simulink model "ROMI_FinalModel"  (R2022b)
settings: Solver=FixedStepDiscrete  StartTime=0.0  StopTime=300  FixedStep=0.1  RelTol=1e-3
libraries: nvidiaAVlib x2, dspindex x2, simulink x2, visiontextngfix x1, deeplib x1, visionstatistics x1
settings Model: Creator=HYUH  LastModifiedBy=HYUH
settings OptimizationCC: StrengthReduction=on  PassReuseOutputArgsAs=Individual arguments  ZeroExternalMemoryAtStartup=off  ZeroInternalMemoryAtStartup=off  InitFltsAndDblsToZero=on  MaxStackSize=64  SimCompilerOptimization=on  OptimizeBlockOrder=speed  OptimizationPriority=Speed  EfficientTunableParamExpr=on
settings DebuggingCC: ParameterTunabilityLossMsg=error
settings HardwareCC: ProdBitPerLong=64  ProdLargestAtomicInteger=LongLong  ProdLargestAtomicFloat=Double  ProdLongLongMode=on  ProdHWDeviceType=ARM Compatible->ARM 64-bit (LP64)  TargetLongLongMode=on
settings ModelReferenceCC: EnableRefExpFcnMdlSchedulingChecks=on
settings SFSimCC: SimHardwareAcceleration=native  SimTargetLang=C++  GPUAcceleration=on  SimDLTargetLibrary=cudnn
settings RTWCC: Description=Embedded Coder  SystemTargetFile=ert.tlc  HardwareBoard=NVIDIA Jetson  TLCOptions="-aInlineSetEventsForThisBaseRateFcn=TLC_FALSE -aSuppressMultiTaskScheduler=TLC_FALSE  -aRateBasedStepFcn=0"  TemplateMakefile=ert_default_tmf  Toolchain=NVCC for NVIDIA Embedded Processors  BuildConfiguration=Faster Runs  TargetLang=C++  GenerateGPUCode=CUDA  DLTargetLibrary=cudnn
settings CodeAppCC: ForceParamTrailComments=on  IgnoreCustomStorageClasses=off  OperatorAnnotations=on  SimulinkDataObjDesc=on  SFDataObjDesc=on  InsertBlockDesc=on
settings ERTTargetCC: MatFileLogging=on  SupportVariableSizeSignals=on  ExtModeStaticAlloc=on  RootIOFormat=Structure reference

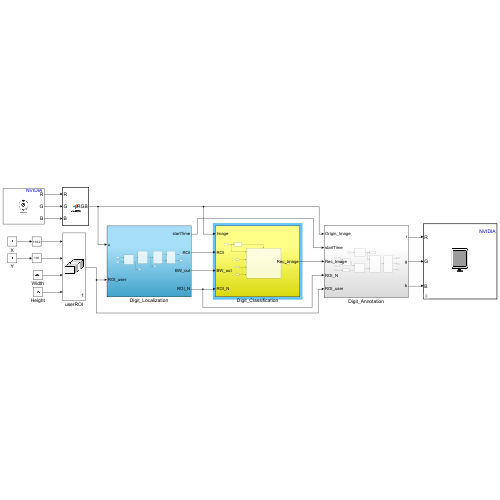
[thumbnail: Simulink's stored preview of the top-level diagram]
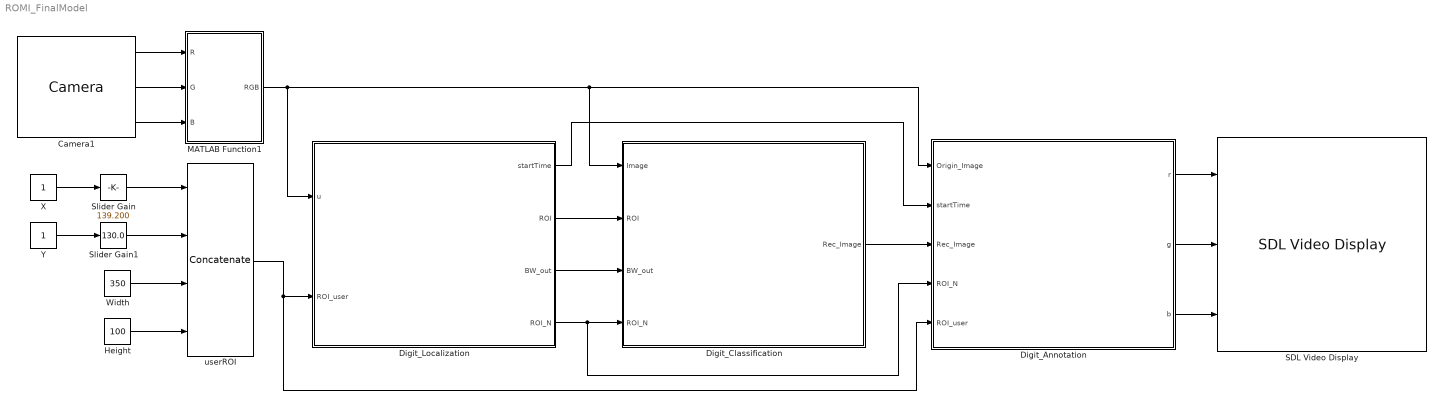
== system ROMI_FinalModel ==
  Camera1 : nvidiaAVlib/Camera  CameraName=UVC Camera (046d:0825)  ImageSize=[640 480]  SampleTime=0.1  SimulateUsing=Code generation
  Digit_Annotation : Subsystem
  Digit_Classification : Subsystem
  Digit_Localization : Subsystem
  Height : Constant  Value=100
  MATLAB Function1 : MATLAB Function  TreatAsAtomicUnit=on
  SDL Video Display : nvidiaAVlib/SDL Video Display  pixelFormat=RGB  pixelOrder=Planar  rowMajor=on  blockPlatform=NVIDIA
  Slider Gain : simulink/Math Operations/Slider Gain  gain=139.200  low=0  high=480
  Slider Gain1 : simulink/Math Operations/Slider Gain  gain=130.0  low=0  high=640
  Width : Constant  Value=350
  X : Constant
  Y : Constant
  userROI : Concatenate  NumInputs=4  Mode=Multidimensional array
  wires:
  Width/1 -> userROI/3
  Height/1 -> userROI/4
  X/1 -> Slider Gain/1
  Y/1 -> Slider Gain1/1
  Camera1/1 -> MATLAB Function1/1(R)
  Camera1/2 -> MATLAB Function1/2(G)
  Camera1/3 -> MATLAB Function1/3(B)
  Slider Gain1/1 -> userROI/2
  Slider Gain/1 -> userROI/1
  MATLAB Function1/1(RGB) -> Digit_Annotation/1(Origin_Image), Digit_Classification/1(Image), Digit_Localization/1(u)
  Digit_Annotation/3(b) -> SDL Video Display/3
  userROI/1 -> Digit_Annotation/5(ROI_user), Digit_Localization/2(ROI_user)
  Digit_Localization/1(startTime) -> Digit_Annotation/2(startTime)
  Digit_Localization/2(ROI) -> Digit_Classification/2(ROI)
  Digit_Localization/3(BW_out) -> Digit_Classification/3(BW_out)
  Digit_Localization/4(ROI_N) -> Digit_Classification/4(ROI_N), Digit_Annotation/4(ROI_N)
  Digit_Classification/1(Rec_Image) -> Digit_Annotation/3(Rec_Image)
  Digit_Annotation/1(r) -> SDL Video Display/1
  Digit_Annotation/2(g) -> SDL Video Display/2

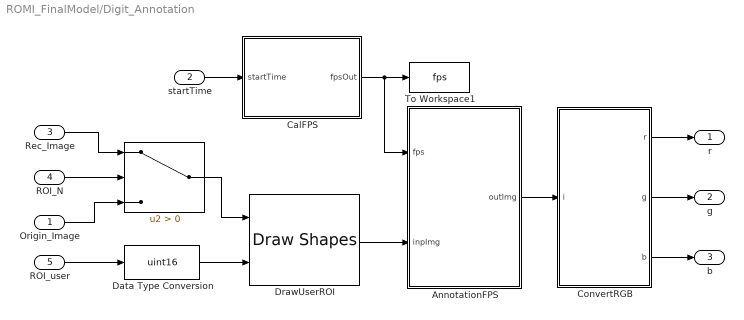
== system ROMI_FinalModel/Digit_Annotation ==
  Origin_Image : Inport
  startTime : Inport  Port=2
  Rec_Image : Inport  Port=3
  ROI_N : Inport  Port=4
  ROI_user : Inport  Port=5
  " " : Switch  Criteria=u2 > Threshold  SaturateOnIntegerOverflow=off  InputSameDT=off
  AnnotationFPS : MATLAB Function  TreatAsAtomicUnit=on
  CalFPS : MATLAB Function  TreatAsAtomicUnit=on
  ConvertRGB : MATLAB Function  TreatAsAtomicUnit=on
  Data Type Conversion : DataTypeConversion  OutDataTypeStr=uint16  SaturateOnIntegerOverflow=off  RndMeth=Floor
  DrawUserROI : visiontextngfix/Draw Shapes  shape=Rectangles  fill=off  lineWidth=3  fillClrSource=Specify via dialog  display=Black  intensity=200  color=[200 255 100]  opacity=0.6  viewport=Entire image  antialiasing=off  inType=Obsolete  imagePorts=One multidimensional signal  roundingMode=Floor  overflowMode=off  memoryMode=Specify word length  memoryWordLength=16  prodOutputMode=Binary point scaling  prodOutputWordLength=32  prodOutputFracLength=14  memoryFracLength=15
  To Workspace1 : ToWorkspace  VariableName=fps  SaveFormat=Structure With Time  SampleTime=-1
  r : Outport
  g : Outport  Port=2
  b : Outport  Port=3
  wires:
  startTime/1 -> CalFPS/1(startTime)
  Rec_Image/1 -> " "/1
  Data Type Conversion/1 -> DrawUserROI/2
  ROI_user/1 -> Data Type Conversion/1
  ROI_N/1 -> " "/2
  Origin_Image/1 -> " "/3
  CalFPS/1(fpsOut) -> To Workspace1/1, AnnotationFPS/1(fps)
  " "/1 -> DrawUserROI/1
  DrawUserROI/1 -> AnnotationFPS/2(inpImg)
  AnnotationFPS/1(outImg) -> ConvertRGB/1(i)
  ConvertRGB/2(g) -> g/1
  ConvertRGB/1(r) -> r/1
  ConvertRGB/3(b) -> b/1

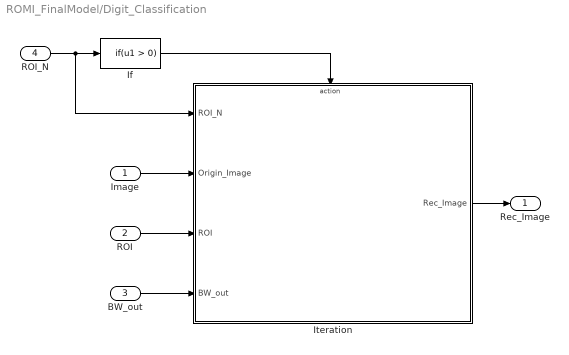
== system ROMI_FinalModel/Digit_Classification ==
  Image : Inport
  ROI : Inport  Port=2
  BW_out : Inport  Port=3
  ROI_N : Inport  Port=4
  If : If  ShowElse=off
  Iteration : Subsystem  TreatAsAtomicUnit=on
  Rec_Image : Outport
  wires:
  Iteration/1(Rec_Image) -> Rec_Image/1
  ROI_N/1 -> If/1, Iteration/1(ROI_N)
  ROI/1 -> Iteration/3(ROI)
  BW_out/1 -> Iteration/4(BW_out)
  Image/1 -> Iteration/2("Origin_Image ")
  If/1 -> Iteration/Action

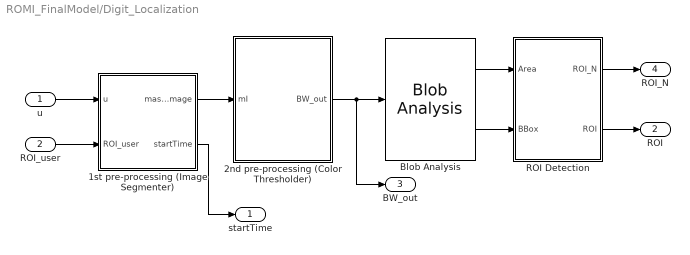
== system ROMI_FinalModel/Digit_Localization ==
  u : Inport
  ROI_user : Inport  Port=2
  1st pre-processing (Image Segmenter) : MATLAB Function  TreatAsAtomicUnit=on
  2nd pre-processing (Color Thresholder) : MATLAB Function  TreatAsAtomicUnit=on
  Blob Analysis : visionstatistics/Blob Analysis  Tag=vipblks_row_conv  area=on  centroid=off  bBox=on  majorAxis=off  minorAxis=off  angle=off  eccentricity=off  equivDiameterSq=off  extent=off  perimeter=off  outDT=double  conn=8  isLabel=off  maxBlobs=50  warnIfNumBlobsExceeded=on  isCount=off  useMinArea=off  minArea=0  useMaxArea=off  maxArea=intmax('uint32')  excludeBorderBlob=off  isOutVarDim=off  isFill=on  fillValues=-1  roundingMode=Floor  overflowMode=off  prodOutputMode=Binary point scaling  prodOutputWordLength=32  prodOutputFracLength=16  accumMode=Binary point scaling  accumWordLength=32  accumFracLength=0  outputMode=Binary point scaling  outputWordLength=32  outputFracLength=16  firstCoeffMode=Binary point scaling  firstCoeffWordLength=16  firstCoeffFracLength=14  secondCoeffMode=Binary point scaling  secondCoeffWordLength=32  secondCoeffFracLength=16
  ROI Detection : MATLAB Function  TreatAsAtomicUnit=on
  startTime : Outport
  ROI : Outport  Port=2
  BW_out : Outport  Port=3
  ROI_N : Outport  Port=4
  wires:
  u/1 -> 1st pre-processing (Image Segmenter)/1(u)
  ROI_user/1 -> 1st pre-processing (Image Segmenter)/2(ROI_user)
  ROI Detection/1(ROI_N) -> ROI_N/1
  Blob Analysis/2 -> ROI Detection/2(BBox)
  2nd pre-processing (Color Thresholder)/1(BW_out) -> BW_out/1, Blob Analysis/1
  1st pre-processing (Image Segmenter)/1(maskedImage) -> 2nd pre-processing (Color Thresholder)/1(mI)
  1st pre-processing (Image Segmenter)/2(startTime) -> startTime/1
  Blob Analysis/1 -> ROI Detection/1(Area)
  ROI Detection/2(ROI) -> ROI/1

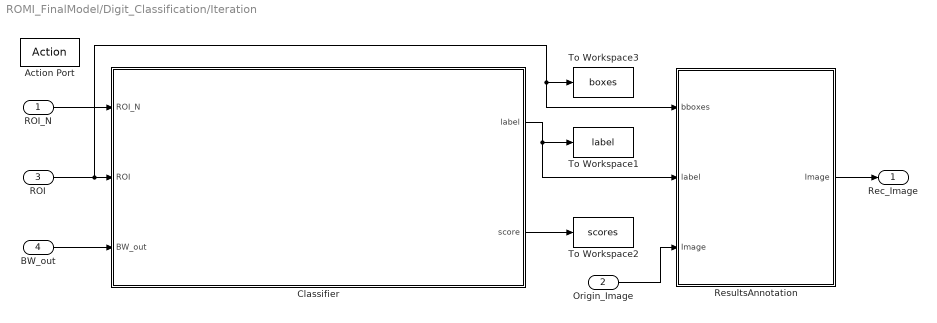
== system ROMI_FinalModel/Digit_Classification/Iteration ==
  ROI_N : Inport
  "Origin_Image " : Inport  Port=2
  ROI : Inport  Port=3
  BW_out : Inport  Port=4
  Action Port : ActionPort  PropagateVarSize=During execution  ActionPortLabel=if(u1 > 0)
  Classifier : Subsystem  TreatAsAtomicUnit=on
  ResultsAnnotation : MATLAB Function  TreatAsAtomicUnit=on
  To Workspace1 : ToWorkspace  VariableName=label  SaveFormat=Structure With Time  SampleTime=-1
  To Workspace2 : ToWorkspace  VariableName=scores  SaveFormat=Structure With Time  SampleTime=-1
  To Workspace3 : ToWorkspace  VariableName=boxes  SaveFormat=Structure With Time  SampleTime=-1
  Rec_Image : Outport
  wires:
  "Origin_Image "/1 -> ResultsAnnotation/3("Image ")
  BW_out/1 -> Classifier/3(BW_out)
  ROI_N/1 -> Classifier/1(ROI_N)
  ROI/1 -> ResultsAnnotation/1(bboxes), To Workspace3/1, Classifier/2(ROI)
  Classifier/1(label) -> ResultsAnnotation/2(label), To Workspace1/1
  Classifier/2(score) -> To Workspace2/1
  ResultsAnnotation/1(Image) -> Rec_Image/1

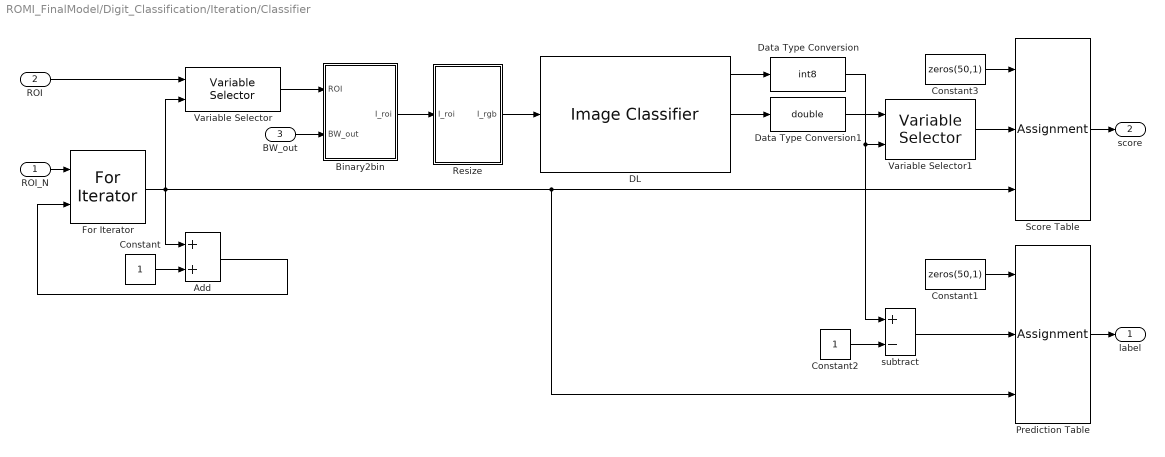
== system ROMI_FinalModel/Digit_Classification/Iteration/Classifier ==
  ROI_N : Inport
  ROI : Inport  Port=2
  BW_out : Inport  Port=3
  Add : Sum
  Binary2bin : MATLAB Function  TreatAsAtomicUnit=on
  Constant : Constant
  Constant1 : Constant  Value=zeros(50,1)
  Constant2 : Constant
  Constant3 : Constant  Value=zeros(50,1)
  DL : deeplib/Image Classifier  Network=Network from MAT-file  NetworkFunction=squeezenet  NetworkFilePath=C:\Users\HYUH\Documents\Paper works\2. [Sensors with HYUH] ROMI\Code\Matlab_Simulink\Deep_alexnet_new_40.mat  MiniBatchSize=128  ResizeInput=on  Classification=on  Predictions=on  ForceInterpretedSim=off  PredictMode=All probabilities and labels  K=5
  Data Type Conversion : DataTypeConversion  OutDataTypeStr=int8  SaturateOnIntegerOverflow=off  RndMeth=Floor
  Data Type Conversion1 : DataTypeConversion  OutDataTypeStr=double  SaturateOnIntegerOverflow=off  RndMeth=Floor
  For Iterator : ForIterator  IterationSource=external  ExternalIncrement=on  IterationVariableDataType=double
  "Prediction Table " : Assignment  DiagnosticForDimensions=Warning  IndexOptions=Index vector (port)  Indices=1  OutputSizes=1
  Resize : MATLAB Function  TreatAsAtomicUnit=on
  "Score Table " : Assignment  DiagnosticForDimensions=Warning  IndexOptions=Index vector (port)  Indices=1  OutputSizes=1
  Variable Selector : dspindex/Variable Selector  NumInputs=1  rowsOrCols=Rows  IdxMode=Variable  Elements=[1 3]  ZerOneIdxMode=One-based  errmode=Clip Index  FillMode=on  FillValues=0
  Variable Selector1 : dspindex/Variable Selector  NumInputs=1  rowsOrCols=Columns  IdxMode=Variable  Elements=[1 3]  ZerOneIdxMode=One-based  errmode=Clip Index  FillMode=on  FillValues=0
  subtract : Sum  Inputs=+-
  label : Outport
  score : Outport  Port=2
  wires:
  subtract/1 -> "Prediction Table "/2
  Constant2/1 -> subtract/2
  Constant/1 -> Add/2
  "Prediction Table "/1 -> label/1
  Constant1/1 -> "Prediction Table "/1
  Resize/1(I_rgb) -> DL/1
  DL/1 -> Data Type Conversion/1
  Binary2bin/1(I_roi) -> Resize/1(I_roi)
  ROI/1 -> Variable Selector/1
  "Score Table "/1 -> score/1
  Constant3/1 -> "Score Table "/1
  Variable Selector1/1 -> "Score Table "/2
  Data Type Conversion1/1 -> Variable Selector1/1
  Add/1 -> For Iterator/2
  Variable Selector/1 -> Binary2bin/1(ROI)
  ROI_N/1 -> For Iterator/1
  BW_out/1 -> Binary2bin/2(BW_out)
  DL/2 -> Data Type Conversion1/1
  Data Type Conversion/1 -> subtract/1, Variable Selector1/2
  For Iterator/1 -> "Score Table "/3, "Prediction Table "/3, Add/1, Variable Selector/2

== matlab function ROMI_FinalModel/Digit_Localization/2nd pre-processing (Color Thresholder) ==
  data: mI input; BW_out output
function BW_out  = prePro2(mI)

RGB = mI;

%%

% Convert RGB image to chosen color space
I = rgb2hsv(RGB);

% Define thresholds for channel 1 based on histogram settings
channel1Min = 0.000;
channel1Max = 1.000;

% Define thresholds for channel 2 based on histogram settings
channel2Min = 0.000;
channel2Max = 0.411;

% Define thresholds for channel 3 based on histogram settings
channel3Min = 0.706;
channel3Max = 1.000;

% Create mask based on chosen histogram thresholds
sliderBW = (I(:,:,1) >= channel1Min ) & (I(:,:,1) <= channel1Max) & ...
    (I(:,:,2) >= channel2Min ) & (I(:,:,2) <= channel2Max) & ...
    (I(:,:,3) >= channel3Min ) & (I(:,:,3) <= channel3Max);
BW = sliderBW;

% Initialize output masked image based on input image.
maskedRGBImage = RGB;

% Set background pixels where BW is false to zero.
maskedRGBImage(repmat(~BW,[1 1 3])) = 0;


% % Convert RGB image to chosen color space
% I = rgb2hsv(RGB);
% 
% % Define thresholds for channel 1 based on histogram settings
% channel1Min = 0.000;
% channel1Max = 1.000;
% 
% % Define thresholds for channel 2 based on histogram settings
% channel2Min = 0.000;
% channel2Max = 0.357;
% 
% % Define thresholds for channel 3 based on histogram settings
% channel3Min = 0.730;
% channel3Max = 1.000;
% 
% % Create mask based on chosen histogram thresholds
% sliderBW = (I(:,:,1) >= channel1Min ) & (I(:,:,1) <= channel1Max) & ...
%     (I(:,:,2) >= channel2Min ) & (I(:,:,2) <= channel2Max) & ...
%     (I(:,:,3) >= channel3Min ) & (I(:,:,3) <= channel3Max);
% BW = sliderBW;
% 
% % Initialize output masked image based on input image.
% maskedRGBImage = RGB;
% 
% % Set background pixels where BW is false to zero.
% maskedRGBImage(repmat(~BW,[1 1 3])) = 0;
%%

% Gray and Binarized Image
I_gray = im2gray(maskedRGBImage);
BinaryMask = imbinarize(I_gray);

%% Additional Pre-processing 

% S = [0 0 0 ;1 1 1 ; 0 0 0];
% maker1 = imerode(BinaryMask, S);
% S = [0 1 0 ;0 1 0 ; 0 1 0];
% maker2 = imerode(maker1, S);
% 
% Iclean = imreconstruct(maker2, BinaryMask);

in_I = BinaryMask;
se = strel('square',2);

% OpenBW : Erode and Dilate (eliminate thin noise)
temp = imerode(in_I,se);
OpenBW = imdilate(temp,se);

% % CloseBW : Dilate and Erode (Fill the hole)
% temp = imdilate(OpenBW,se);
% CloseBW = imerode(temp,se);

squareBW = imdilate(OpenBW, se);

% erodBW1 = imerode(squareBW,strel('line',10,0));
% erodBW2 = imerode(erodBW1, strel('line',10,90));

% se = strel('square',5);
% dilateBW32 = uint32(dilateBW);
% closeBW = imclose(dilateBW32,se);
% figure, imshow(closeBW)

BW_out = squareBW;
end

== matlab function ROMI_FinalModel/Digit_Localization/ROI Detection ==
  data: ROI_N output; Area input; BBox input; ROI output
function [ROI_N, ROI]  = roiDetection(Area, BBox)

    ROI = zeros(size(BBox,1), size(BBox,2));
    areaConstraint = Area > 150;

    % Keep regions that meet the area constraint.
    roi = double(BBox(areaConstraint, :));

    % Compute the aspect ratio.
    width  = roi(:,3);
    height = roi(:,4);
    aspectRatio = width ./ height;
    
    % An aspect ratio between 0.25 and 1 is typical for individual characters
    % as they are usually not very short and wide or very tall and skinny.
    roi = roi( aspectRatio > 0.3 & aspectRatio < 0.8 ,:);
    
    ROI_N = size(roi,1);
    ROI(1:ROI_N,:) = roi;

end

== matlab function ROMI_FinalModel/MATLAB Function1 ==
  data: R input; RGB output; G input; B input
function RGB  = rgb2Img(R,G,B)
RGB = coder.nullcopy(uint8(zeros(size(R,1),size(R,2),3)));
RGB(:,:,1) = R;
RGB(:,:,2) = G;
RGB(:,:,3) = B;
end

== matlab function ROMI_FinalModel/Digit_Annotation/CalFPS ==
  data: startTime input; fpsOut output
function fpsOut  = calcFPS(startTime)
finishTime = datetime;

diffTime = seconds(finishTime-datetime(startTime));
persistent count;
if isempty(count)
    count = 0;
end
persistent fps;
if isempty(fps)
    fps = 0;
end
fps = (count*fps + 1*(1/diffTime))/(count+1);

count = count + 1;
fpsOut = fps;

== matlab function ROMI_FinalModel/Digit_Classification/Iteration/Classifier/Binary2bin ==
  data: ROI input; BW_out input; I_roi output size=28, 28
function I_roi  = binROI(ROI,BW_out)

% Crop the image based on the area of interest
bin = imcrop(BW_out, ROI);

% %I_roi = coder.nullcopy(zeros(28,28,'logical'));
% I_roi = imresize(bin, [28 28]);

I_padd = padarray(bin,[floor((max(size(bin))-size(bin,1))/2),floor((max(size(bin))-size(bin,2))/2)],0,'both');
I_roi = imresize(I_padd, [28 28]);
I_roi = imcomplement(I_roi);

== matlab function ROMI_FinalModel/Digit_Classification/Iteration/ResultsAnnotation ==
  data: bboxes input; label input; Image input; Image output
function Image = annoImg( bboxes, label, Image)
        Image = insertObjectAnnotation(Image, 'rectangle',bboxes,label);
end

== matlab function ROMI_FinalModel/Digit_Localization/1st pre-processing (Image Segmenter) ==
  data: u input; maskedImage output; ROI_user input; startTime output
function [maskedImage, startTime]  = prePro1(u, ROI_user)

currentTime = datetime;
startTime = [currentTime.Year currentTime.Month currentTime.Day currentTime.Hour ...
    currentTime.Minute currentTime.Second];

% Convert RGB image into L*a*b* color space.
X = rgb2lab(u);

% Create empty mask.
BW = false(size(X,1),size(X,2));

% ROI 그리기

xPos = [ROI_user(1), ROI_user(1), ROI_user(1)+ROI_user(3), ROI_user(1)+ROI_user(3)];
yPos = [ROI_user(2), ROI_user(2)+ROI_user(4), ROI_user(2)+ROI_user(4), ROI_user(2)];

%ROI_user = [xPos(1), yPos(1), ROI_width, ROI_height];
%ROI_width = xPos(3)-xPos(2);
%ROI_height = yPos(2)-yPos(1);
%xPos = [181.5065 181.5065 475.2642 475.2642];
%yPos = [247.2758 309.4262 309.4262 247.2758];

m = size(BW, 1);
n = size(BW, 2);
addedRegion = poly2mask(xPos, yPos, m, n);
BW = BW | addedRegion;

% Create masked image.
maskedImage = u;
maskedImage(repmat(~BW,[1 1 3])) = 0;

end

== matlab function ROMI_FinalModel/Digit_Classification/Iteration/Classifier/Resize ==
  data: I_roi input; I_rgb output
function I_rgb = reSize(I_roi)

%I_roi = coder.nullcopy(zeros(28,28,'logical'));W
I = im2uint8(imresize(I_roi,[227, 227]));
I_rgb = cat(3, I, I, I);

== matlab function ROMI_FinalModel/Digit_Annotation/ConvertRGB ==
  data: i input; r output; g output; b output
function [r,g,b] = ImageToRGB(i)
%#codegen
r = rot90(flip(i(:,:,1),2));
g = rot90(flip(i(:,:,2),2));
b = rot90(flip(i(:,:,3),2));
end

== matlab function ROMI_FinalModel/Digit_Annotation/AnnotationFPS ==
  data: fps input; inpImg input; outImg output
function outImg = insertFPS(fps, inpImg)


%% Insert prediction with scores in the image

%Pad Image
%outImg = padarray(inpImg,[0,100],0,'pre');

outImg = insertText(inpImg, [10 80],['FPS : ' sprintf('%0.2f',fps) ], 'AnchorPoint','LeftBottom');
